simulink model "SelfBalancingRobot"  (R2017a)
settings: Solver=VariableStepAuto  StartTime=0.0  StopTime=10.0  RelTol=1e-3
values from neighbouring files (symbols this model uses):
  K1 = -119.0071    [pendcartsim.m]
  K2 = 1.402    [Stepper_Model_2017_10_31_Script.m]    (also in pendcartsim.m = 0.0402)
  p = 5.4277    [pendcartsim.m]
  p1 = 25.4277    [pendcartsim.m]
  theta0 = 5*pi/180    (= 0.0872664625997)    [Stepper_Model_2017_10_31_Script.m]    (also in pendcartsim.m)
settings Model: Creator=Administrator  LastModifiedBy=Administrator

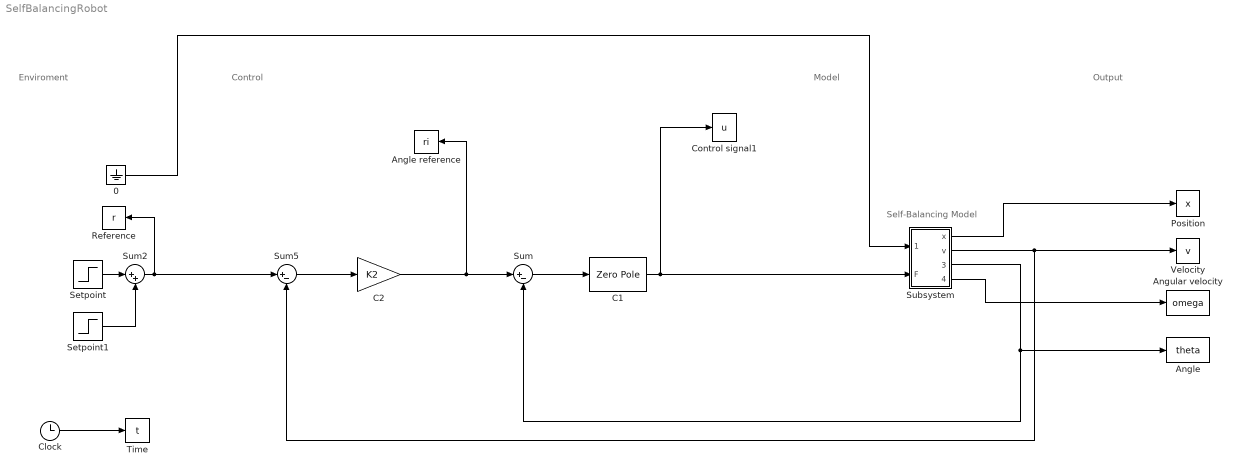
== system SelfBalancingRobot ==
  note: Model
  note: Self-Balancing Model
  note: Output
  note: Control
  note: Enviroment
  0 : Ground
  Angle : ToWorkspace  VariableName=theta  SampleTime=-1
  Angle reference : ToWorkspace  VariableName=ri  SampleTime=-1
  Angular velocity : ToWorkspace  VariableName=omega  SampleTime=-1
  C1 : ZeroPole  Zeros=[-p]  Poles=[-p1]  Gain=[K1]
  C2 : Gain  Gain=K2
  Clock : Clock
  Control signal1 : ToWorkspace  VariableName=u  SampleTime=-1
  Position : ToWorkspace  VariableName=x  SampleTime=-1
  Reference : ToWorkspace  VariableName=r  SampleTime=-1
  Setpoint : Step  Time=10  After=0.5  SampleTime=0
  Setpoint1 : Step  Time=20  After=-0.5  SampleTime=0
  Subsystem : Subsystem
  Sum : Sum  Inputs=|+-
  Sum2 : Sum  Inputs=|++
  Sum5 : Sum  Inputs=|+-
  Time : ToWorkspace  VariableName=t  SampleTime=-1
  Velocity : ToWorkspace  VariableName=v  SampleTime=-1
  wires:
  0/1 -> Subsystem/1(alpha)
  C2/1 -> Angle reference/1, Sum/1
  Setpoint1/1 -> Sum2/2
  Setpoint/1 -> Sum2/1
  Subsystem/3(theta) -> Angle/1, Sum/2
  Subsystem/2(v) -> Velocity/1, Sum5/2
  Subsystem/4(omega) -> Angular velocity/1
  C1/1 -> Subsystem/2(F), Control signal1/1
  Sum2/1 -> Sum5/1, Reference/1
  Sum/1 -> C1/1
  Sum5/1 -> C2/1
  Subsystem/1(x) -> Position/1
  Clock/1 -> Time/1

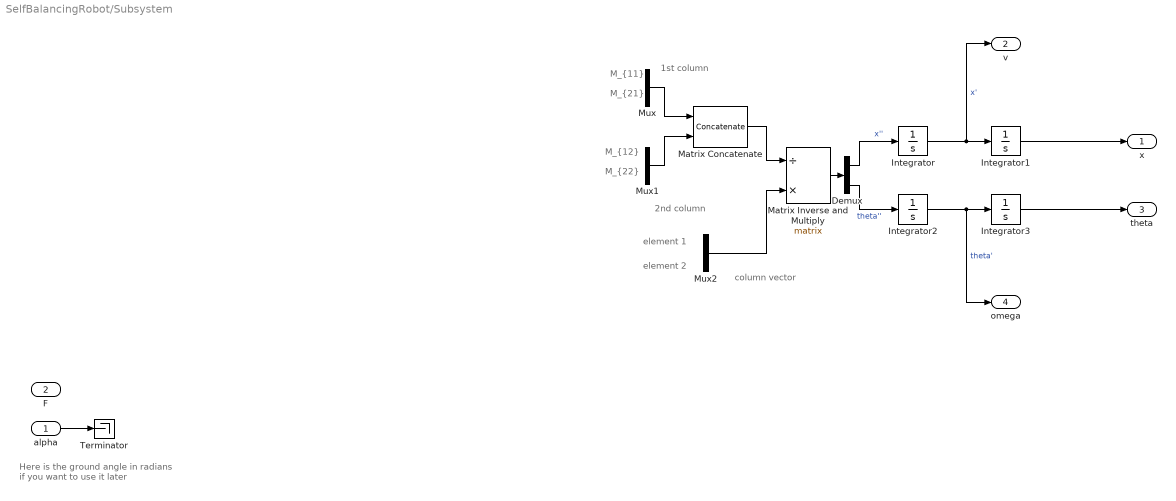
== system SelfBalancingRobot/Subsystem ==
  note: Here is the ground angle in
      | radians if you want to use it later
  note: M_{12}
  note: M_{21}
  note: element 1
  note: M_{22}
  note: M_{11}
  note: element 2
  note: 2nd column
  note: column vector
  note: 1st column
  alpha : Inport
  F : Inport  Port=2
  Demux : Demux  Outputs=2
  Integrator : Integrator
  Integrator1 : Integrator
  Integrator2 : Integrator
  Integrator3 : Integrator  InitialCondition=theta0
  Matrix Concatenate : Concatenate  Mode=Multidimensional array  ConcatenateDimension=2
  Matrix Inverse and Multiply : Product  Inputs=/*  Multiplication=Matrix(*)
  Mux : Mux  Inputs=2
  Mux1 : Mux  Inputs=2
  Mux2 : Mux  Inputs=2
  Terminator : Terminator
  x : Outport
  v : Outport  Port=2
  theta : Outport  Port=3
  omega : Outport  Port=4
  wires:
  Integrator/1 -> Integrator1/1, v/1  "x'"
  Mux2/1 -> Matrix Inverse and Multiply/2
  Demux/1 -> Integrator/1  "x''"
  Integrator3/1 -> theta/1
  Matrix Inverse and Multiply/1 -> Demux/1
  Demux/2 -> Integrator2/1  "theta''"
  Mux/1 -> Matrix Concatenate/1
  Integrator2/1 -> Integrator3/1, omega/1  "theta'"
  Mux1/1 -> Matrix Concatenate/2
  Integrator1/1 -> x/1
  alpha/1 -> Terminator/1
  Matrix Concatenate/1 -> Matrix Inverse and Multiply/1
